simulink model "CaptureOutputs_compatible"  (R2017b)
settings: Solver=ode4  StartTime=0.0  StopTime=SimEndTime  FixedStep=TimeStep  RelTol=1e-3
undefined symbols (not defined in the file or in its folder): SampleTime
settings Model: Creator=Ethan  LastModifiedBy=Ethan
settings ModelReferenceCC: ModelReferenceNumInstancesAllowed=Single
settings SFSimCC: SimUseLocalCustomCode=on
settings RTWCC: RTWUseLocalCustomCode=on

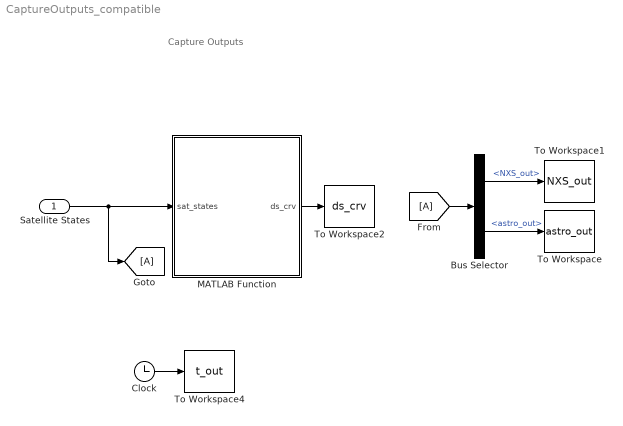
== system CaptureOutputs_compatible ==
  note: Capture Outputs
  Satellite States : Inport  OutDataTypeStr=Bus: Bus_outputs
  Bus Selector : BusSelector  OutputSignals=NXS_out,astro_out
  Clock : Clock
  MATLAB Function : MATLAB Function  TreatAsAtomicUnit=on
  To Workspace : ToWorkspace  VariableName=astro_out  SampleTime=SampleTime
      settings: Save2DSignal=2-D array (concatenate along first dimension)
  To Workspace1 : ToWorkspace  VariableName=NXS_out  SampleTime=SampleTime
      settings: Save2DSignal=2-D array (concatenate along first dimension)
  To Workspace2 : ToWorkspace  VariableName=ds_crv  SampleTime=SampleTime
      settings: Save2DSignal=2-D array (concatenate along first dimension)
  To Workspace4 : ToWorkspace  VariableName=t_out  SampleTime=SampleTime
      settings: Save2DSignal=2-D array (concatenate along first dimension)
  wires:
  Satellite States/1 -> [A], MATLAB Function/1(sat_states)
  MATLAB Function/1(ds_crv) -> To Workspace2/1
  [A] -> Bus Selector/1
  Bus Selector/2 -> To Workspace/1  "<astro_out>"
  Bus Selector/1 -> To Workspace1/1  "<NXS_out>"
  Clock/1 -> To Workspace4/1

== matlab function CaptureOutputs_compatible/MATLAB Function ==
  data: sat_states input; ds_crv output
function ds_crv  = i2relRTN(sat_states)

NXS = sat_states.NXS_out;
R = norm(NXS.r_i);
astro = sat_states.astro_out;

i2lvlh = rv2RTN(NXS.r_i, NXS.v_i);

rel_state_lvlh = states_i2lvlh(NXS, astro);
dx = rel_state_lvlh(1);
dy = rel_state_lvlh(2);
dz = rel_state_lvlh(3);

dx_dot = rel_state_lvlh(4);
dy_dot = rel_state_lvlh(5);
dz_dot = rel_state_lvlh(6);

R1 = norm([R + dx ; dy; dz]);

ds_crv = zeros(6, 1);


phi = atan2(dy, R + dx);
psi = asin(dz / R1);

ds_crv(1) = R1 - R;
ds_crv(2) = R * phi;
ds_crv(3) = R * psi;

R_dot = (i2lvlh * NXS.v_i)' * (i2lvlh * NXS.r_i) / R;
R1_dot = sqrt((R_dot + dx_dot)^2 + dy_dot^2 + dz_dot^2);

phi_dot = (dy_dot * (R + dx) - dy * (R_dot + dx_dot)) / ...
    (dy^2 + (R + dx)^2);
psi_dot = (dz_dot*R1 - dz * R1_dot) / R1^2 * sqrt(1 + (dz^2 / (dy^2 + (R + dx)^2)));

ds_crv(4) = R1_dot - R_dot;
ds_crv(5) = R_dot * phi + R * phi_dot;
ds_crv(6) = R_dot * psi + R * psi_dot;
end
